simulink library "simetran"  (R2024b)
settings: Solver=VariableStepAuto  StartTime=0.0  StopTime=10.0  RelTol=1e-3
undefined symbols (not defined in the file): Csnu, gcbh, h, ResistanceM, Rsnu, Rt4, sps_rtmsupport, Ti, Ts, Z, Zm
libraries: fl_lib x81, nesl_utility x48, ee_lib x23
(part 2 of 3)

== system simetran/MATE_SSE_3Level/Subsystem2 ==
  g : Inport
  Capacitor : fl_lib/Electrical/Electrical Elements/Capacitor  c=SnubberCapacitance F  r=0 Ohm  g=0 1/Ohm  i_specify=off  i_priority=None  i=0 A  i_nominal_specify=off  i_nominal_value=1  i_nominal_unit=A  v_specify=off  v_priority=None  v=0 V  v_nominal_specify=off  v_nominal_value=1  v_nominal_unit=V  vc_specify=off  vc_priority=High  vc=0 V  vc_nominal_specify=off  vc_nominal_value=1  vc_nominal_unit=V
  Resistor : fl_lib/Electrical/Electrical Elements/Resistor  R=SnubberResistance Ohm  i_specify=off  i_priority=None  i=0 A  i_nominal_specify=off  i_nominal_value=1  i_nominal_unit=A  v_specify=off  v_priority=None  v=0 V  v_nominal_specify=off  v_nominal_value=1  v_nominal_unit=V
  SPST Switch : ee_lib/Switches & Breakers/SPST Switch  R_closed=Ron*2 Ohm  G_open=1e-6 S  Threshold=0.5 V  Width=0 V  model_dynamics=0  t_on=1e-3 s  t_off=1e-3 s  initial_vT=0 V
      settings: InternalSimscapePortConfiguration="{\"Bottom\":[],\"Left\":[{\"id\":\"vT\",\"label\":\"vT\",\"type\":\"input\"},{\"id\":\"p\",\"label\":\"\",\"type\":\"foundation.electrical.electrical\"}],\"Right\":[{\"id\":\"n\",\"label\":\"\",\"type\":\"foundation.electrical.electrical\"}],\"Top\":[]}"
  Simulink-PS Converter : nesl_utility/Simulink-PS Converter  PhysicalDomain=network_engine_domain  SubClassName=ps_input  LeftPortType=input  RightPortType=output  PseudoPeriodic=off  Frequencies=[]  NoiseDistribution=none  NoiseParameters=[]  Unit=1  AffineConversion=off  FilteringAndDerivatives=provide  SimscapeFilterOrder=1  InputFilterTimeConstant=0.001  UdotUserProvided=0
  P : PMIOPort  Side=Left
  N : PMIOPort  Port=2  Side=Right
  wires:
  g/1 -> Simulink-PS Converter/1
  connections:
  Capacitor/RConn1 -- Resistor/LConn1
  N/RConn1 -- Resistor/RConn1 -- SPST Switch/RConn1
  Simulink-PS Converter/RConn1 -- SPST Switch/LConn1
  P/RConn1 -- Capacitor/LConn1 -- SPST Switch/LConn2

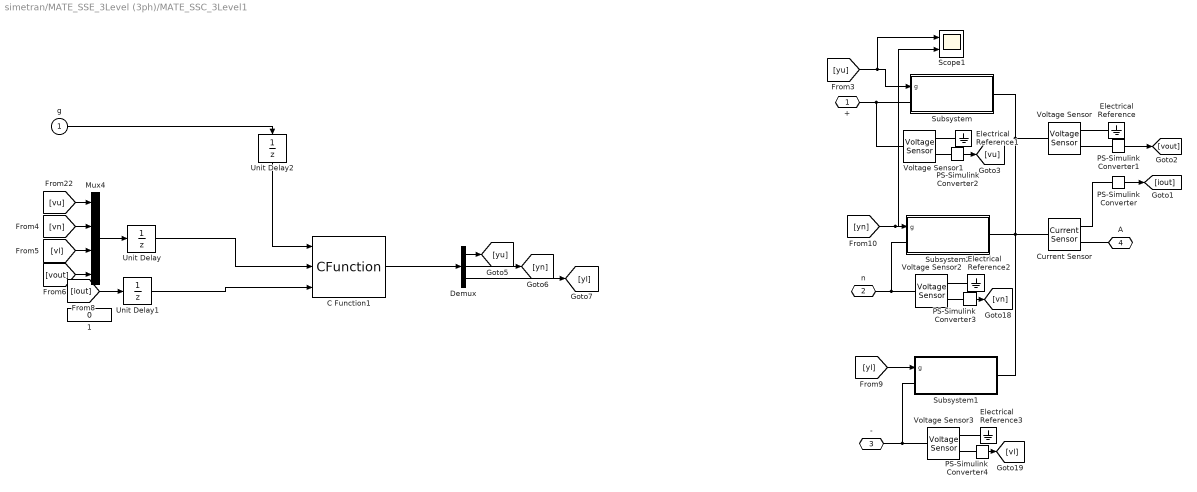
== system simetran/MATE_SSE_3Level (3ph)/MATE_SSC_3Level1 ==
  g : Inport
  1 : Constant  Value=0
  C Function1 : CFunction  OutputCode=|  InitializeConditionsCode=status_old=0;  CodegenOutputCode=|  CodegenInitializeConditionsCode=status_old=0;  CustomCodeSettingLocation=ModelConfigurationParameters
      OutputCode=|
      | {
      |     double status;
      | 
      |     //InputRealPtrsType gg      = ssGetInputPortRealSignalPtrs(S,0);
      |     //InputRealPtrsType Vtermm  = ssGetInputPortRealSignalPtrs(S,1);
      |     //InputRealPtrsType ioutt   = ssGetInputPortRealSignalPtrs(S,2);
      |     //InputRealPtrsType tol     = ssGetInputPortRealSignalPtrs(S,3);
      | 
      | 
      |     //real_T            *sw       =  ssGetOutputPortRealSignal(S,0);  // sw
      |     //real_T			  *stat     =  ssGetOutputPortRealSignal(S,1);  // status
      | 
      | 
      | 
      |     //mexPrintf("OUTPUTpause:\n");
      |     //mexEvalString("pause(2);");
      | 
      | 
      | 
      |     //real_T *status_old    = (real_T*) ssGetDWork(S,0);
      |     //real_T status[1];
      | 
      | 
      |     //real_T  g[4];
      |     //real_T  Vterm[4];
      |  
      | 
      |     //real_T iout[1];
      | 
      |    // *(g+0)= *gg[0];
      |    // *(g+1)= *gg[1];
      |    // *(g+2)= *gg[2];
      |    // *(g+3)= *gg[3];
      | 
      |    // *(Vterm+0)= *Vtermm[0];
      |    // *(Vterm+1)= *Vtermm[1];
      |    // *(Vterm+2)= *Vtermm[2];
      |    // *(Vterm+3)= *Vtermm[3];
      | 
      |    // iout= *ioutt[0];
      | 
      | 
      |  
      | 
      | 
      |     if (*(g+0)>0.5 && *(g+1)>0.5) {
      |         *(sw+0)=1;*(sw+1)=0;*(sw+2)=0;status=1;
      |     }
      |     else if (*(g+2)>0.5  && *(g+3)>0.5) {
      |         *(sw+0)=0;*(sw+1)=0;*(sw+2)=1;status=2;
      |     }
      |     else if (*(g+1)>0.5  && *(g+2)>0.5) {
      |         *(sw+0)=0;*(sw+1)=1;*(sw+2)=0;status=3;
      |     }
      |     else if (*(g+1)>0.5 && iout>0) {
      |         *(sw+0)=0;*(sw+1)=1;*(sw+2)=0;status=4;
      |     }
      |     else if (*(g+2)>0.5 && iout<0) {
      |         *(sw+0)=0;*(sw+1)=1;*(sw+2)=0;status=5;
      |     }
      |     else if ( (iout>0 && status_old<=6)) { //|| (*(iout>tol[0] && status_old>5) )  {
      |         *(sw+0)=0;*(sw+1)=0;*(sw+2)=1;status=6;
      |     }
      |     else if ( (iout<0 && status_old<=5) || (iout<0 && status_old==7) ) { // || (iout<(0-tol[0]) && status_old[0]>5)   ) {
      |         *(sw+0)=1;*(sw+1)=0;*(sw+2)=0;status=7;
      |     }
      |     else if ( (*(Vterm+3)>*(Vterm+1) && *(g+2)>0.5) || (*(Vterm+3)<*(Vterm+1)  && *(g+1)>0.5) ) {
      |         *(sw+0)=0;*(sw+1)=1;*(sw+2)=0;status=8;
      |     }
      |     else if (*(Vterm+3)>*(Vterm+0)) {
      |         *(sw+0)=1;*(sw+1)=0;*(sw+2)=0;status=9;
      |     }
      |     else if (*(Vterm+3)<*(Vterm+2)) {
      |         *(sw+0)=0;*(sw+1)=0;*(sw+2)=1;status=10;
      |     }
      |     else {
      |         *(sw+0)=0;*(sw+1)=0;*(sw+2)=0;status=11;
      |     }
      | 
      | 
      | 
      |     status_old=status;
      | 
      | 
      | }
      CodegenOutputCode=|
      | {
      |     double status;
      | 
      |     //InputRealPtrsType gg      = ssGetInputPortRealSignalPtrs(S,0);
      |     //InputRealPtrsType Vtermm  = ssGetInputPortRealSignalPtrs(S,1);
      |     //InputRealPtrsType ioutt   = ssGetInputPortRealSignalPtrs(S,2);
      |     //InputRealPtrsType tol     = ssGetInputPortRealSignalPtrs(S,3);
      | 
      | 
      |     //real_T            *sw       =  ssGetOutputPortRealSignal(S,0);  // sw
      |     //real_T			  *stat     =  ssGetOutputPortRealSignal(S,1);  // status
      | 
      | 
      | 
      |     //mexPrintf("OUTPUTpause:\n");
      |     //mexEvalString("pause(2);");
      | 
      | 
      | 
      |     //real_T *status_old    = (real_T*) ssGetDWork(S,0);
      |     //real_T status[1];
      | 
      | 
      |     //real_T  g[4];
      |     //real_T  Vterm[4];
      |  
      | 
      |     //real_T iout[1];
      | 
      |    // *(g+0)= *gg[0];
      |    // *(g+1)= *gg[1];
      |    // *(g+2)= *gg[2];
      |    // *(g+3)= *gg[3];
      | 
      |    // *(Vterm+0)= *Vtermm[0];
      |    // *(Vterm+1)= *Vtermm[1];
      |    // *(Vterm+2)= *Vtermm[2];
      |    // *(Vterm+3)= *Vtermm[3];
      | 
      |    // iout= *ioutt[0];
      | 
      | 
      |  
      | 
      | 
      |     if (*(g+0)>0.5 && *(g+1)>0.5) {
      |         *(sw+0)=1;*(sw+1)=0;*(sw+2)=0;status=1;
      |     }
      |     else if (*(g+2)>0.5  && *(g+3)>0.5) {
      |         *(sw+0)=0;*(sw+1)=0;*(sw+2)=1;status=2;
      |     }
      |     else if (*(g+1)>0.5  && *(g+2)>0.5) {
      |         *(sw+0)=0;*(sw+1)=1;*(sw+2)=0;status=3;
      |     }
      |     else if (*(g+1)>0.5 && iout>0) {
      |         *(sw+0)=0;*(sw+1)=1;*(sw+2)=0;status=4;
      |     }
      |     else if (*(g+2)>0.5 && iout<0) {
      |         *(sw+0)=0;*(sw+1)=1;*(sw+2)=0;status=5;
      |     }
      |     else if ( (iout>0 && status_old<=6)) { //|| (*(iout>tol[0] && status_old>5) )  {
      |         *(sw+0)=0;*(sw+1)=0;*(sw+2)=1;status=6;
      |     }
      |     else if ( (iout<0 && status_old<=5) || (iout<0 && status_old==7) ) { // || (iout<(0-tol[0]) && status_old[0]>5)   ) {
      |         *(sw+0)=1;*(sw+1)=0;*(sw+2)=0;status=7;
      |     }
      |     else if ( (*(Vterm+3)>*(Vterm+1) && *(g+2)>0.5) || (*(Vterm+3)<*(Vterm+1)  && *(g+1)>0.5) ) {
      |         *(sw+0)=0;*(sw+1)=1;*(sw+2)=0;status=8;
      |     }
      |     else if (*(Vterm+3)>*(Vterm+0)) {
      |         *(sw+0)=1;*(sw+1)=0;*(sw+2)=0;status=9;
      |     }
      |     else if (*(Vterm+3)<*(Vterm+2)) {
      |         *(sw+0)=0;*(sw+1)=0;*(sw+2)=1;status=10;
      |     }
      |     else {
      |         *(sw+0)=0;*(sw+1)=0;*(sw+2)=0;status=11;
      |     }
      | 
      | 
      | 
      |     status_old=status;
      | 
      | 
      | }
  Current Sensor : fl_lib/Electrical/Electrical Sensors/Current Sensor
  Demux : Demux  Outputs=3
  Electrical Reference{,1..3} (4 alike) : fl_lib/Electrical/Electrical Elements/Electrical Reference
  Mux4 : Mux
  PS-Simulink Converter{,1..4} (5 alike) : nesl_utility/PS-Simulink Converter  PhysicalDomain=network_engine_domain  SubClassName=ps_output  LeftPortType=input  RightPortType=output  PseudoPeriodic=off  Frequencies=[]  VectorFormat=inherit  Unit=inherit  AffineConversion=off
  Scope1 : Scope  NumInputPorts=2
  Subsystem : Subsystem
  Subsystem1 : Subsystem
  Subsystem2 : Subsystem
  Unit Delay : UnitDelay  SampleTime=Ts  HasFrameUpgradeWarning=on
  Unit Delay1 : UnitDelay  SampleTime=Ts  HasFrameUpgradeWarning=on
  Unit Delay2 : UnitDelay  SampleTime=Ts  HasFrameUpgradeWarning=on
  Voltage Sensor{,1..3} (4 alike) : fl_lib/Electrical/Electrical Sensors/Voltage Sensor
  + : PMIOPort  Side=Left
  n : PMIOPort  Port=2  Side=Left
  - : PMIOPort  Port=3  Side=Left
  A : PMIOPort  Port=4  Side=Right
  wires:
  Mux4/1 -> Unit Delay/1
  Demux/2 -> [yn]
  [vu] -> Mux4/1
  [vn] -> Mux4/2
  [vl] -> Mux4/3
  [vout] -> Mux4/4
  g/1 -> Unit Delay2/1
  Demux/3 -> [yl]
  Demux/1 -> [yu]
  [yu] -> Scope1/1, Subsystem/1(g)
  [yl] -> Subsystem1/1(g)
  [yn] -> Subsystem2/1(g), Scope1/2
  PS-Simulink Converter/1 -> [iout]
  PS-Simulink Converter1/1 -> [vout]
  PS-Simulink Converter2/1 -> [vu]
  PS-Simulink Converter3/1 -> [vn]
  PS-Simulink Converter4/1 -> [vl]
  [iout] -> Unit Delay1/1
  C Function1/1 -> Demux/1
  Unit Delay/1 -> C Function1/2
  Unit Delay1/1 -> C Function1/3
  Unit Delay2/1 -> C Function1/1
  connections:
  +/RConn1 -- Subsystem/LConn1 -- Voltage Sensor1/LConn1
  -/RConn1 -- Subsystem1/LConn1 -- Voltage Sensor3/LConn1
  Current Sensor/LConn1 -- Subsystem1/RConn1 -- Subsystem2/RConn1 -- Subsystem/RConn1 -- Voltage Sensor/LConn1
  n/RConn1 -- Subsystem2/LConn1 -- Voltage Sensor2/LConn1
  A/RConn1 -- Current Sensor/RConn2
  PS-Simulink Converter/LConn1 -- Current Sensor/RConn1
  Voltage Sensor/RConn2 -- Electrical Reference/LConn1
  Voltage Sensor/RConn1 -- PS-Simulink Converter1/LConn1
  Voltage Sensor1/RConn2 -- Electrical Reference1/LConn1
  Voltage Sensor1/RConn1 -- PS-Simulink Converter2/LConn1
  Voltage Sensor2/RConn1 -- PS-Simulink Converter3/LConn1
  Voltage Sensor2/RConn2 -- Electrical Reference2/LConn1
  Voltage Sensor3/RConn2 -- Electrical Reference3/LConn1
  Voltage Sensor3/RConn1 -- PS-Simulink Converter4/LConn1

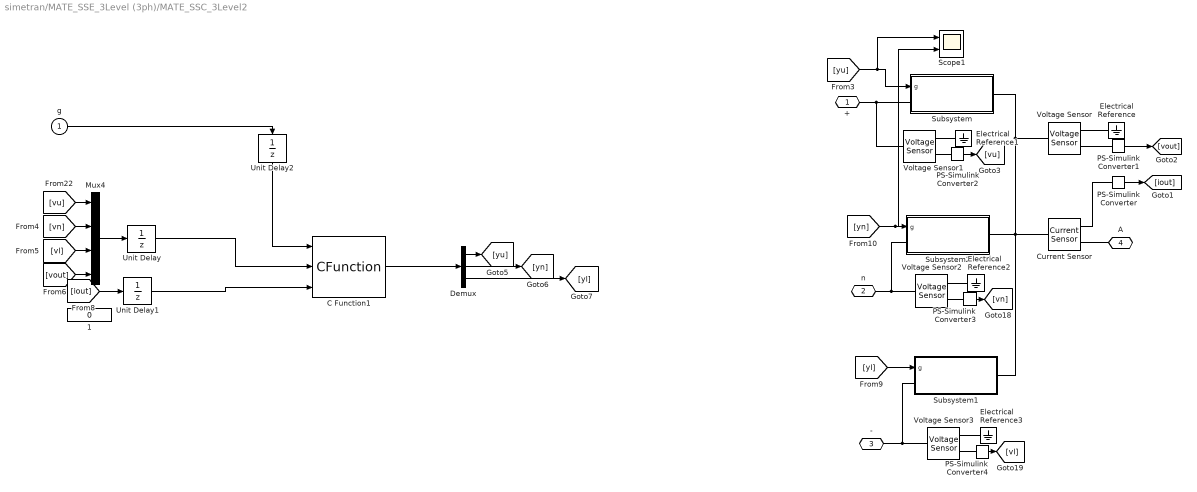
== system simetran/MATE_SSE_3Level (3ph)/MATE_SSC_3Level2 ==
  g : Inport
  1 : Constant  Value=0
  C Function1 : CFunction  OutputCode=|  InitializeConditionsCode=status_old=0;  CodegenOutputCode=|  CodegenInitializeConditionsCode=status_old=0;  CustomCodeSettingLocation=ModelConfigurationParameters
      OutputCode=|
      | {
      |     double status;
      | 
      |     //InputRealPtrsType gg      = ssGetInputPortRealSignalPtrs(S,0);
      |     //InputRealPtrsType Vtermm  = ssGetInputPortRealSignalPtrs(S,1);
      |     //InputRealPtrsType ioutt   = ssGetInputPortRealSignalPtrs(S,2);
      |     //InputRealPtrsType tol     = ssGetInputPortRealSignalPtrs(S,3);
      | 
      | 
      |     //real_T            *sw       =  ssGetOutputPortRealSignal(S,0);  // sw
      |     //real_T			  *stat     =  ssGetOutputPortRealSignal(S,1);  // status
      | 
      | 
      | 
      |     //mexPrintf("OUTPUTpause:\n");
      |     //mexEvalString("pause(2);");
      | 
      | 
      | 
      |     //real_T *status_old    = (real_T*) ssGetDWork(S,0);
      |     //real_T status[1];
      | 
      | 
      |     //real_T  g[4];
      |     //real_T  Vterm[4];
      |  
      | 
      |     //real_T iout[1];
      | 
      |    // *(g+0)= *gg[0];
      |    // *(g+1)= *gg[1];
      |    // *(g+2)= *gg[2];
      |    // *(g+3)= *gg[3];
      | 
      |    // *(Vterm+0)= *Vtermm[0];
      |    // *(Vterm+1)= *Vtermm[1];
      |    // *(Vterm+2)= *Vtermm[2];
      |    // *(Vterm+3)= *Vtermm[3];
      | 
      |    // iout= *ioutt[0];
      | 
      | 
      |  
      | 
      | 
      |     if (*(g+0)>0.5 && *(g+1)>0.5) {
      |         *(sw+0)=1;*(sw+1)=0;*(sw+2)=0;status=1;
      |     }
      |     else if (*(g+2)>0.5  && *(g+3)>0.5) {
      |         *(sw+0)=0;*(sw+1)=0;*(sw+2)=1;status=2;
      |     }
      |     else if (*(g+1)>0.5  && *(g+2)>0.5) {
      |         *(sw+0)=0;*(sw+1)=1;*(sw+2)=0;status=3;
      |     }
      |     else if (*(g+1)>0.5 && iout>0) {
      |         *(sw+0)=0;*(sw+1)=1;*(sw+2)=0;status=4;
      |     }
      |     else if (*(g+2)>0.5 && iout<0) {
      |         *(sw+0)=0;*(sw+1)=1;*(sw+2)=0;status=5;
      |     }
      |     else if ( (iout>0 && status_old<=6)) { //|| (*(iout>tol[0] && status_old>5) )  {
      |         *(sw+0)=0;*(sw+1)=0;*(sw+2)=1;status=6;
      |     }
      |     else if ( (iout<0 && status_old<=5) || (iout<0 && status_old==7) ) { // || (iout<(0-tol[0]) && status_old[0]>5)   ) {
      |         *(sw+0)=1;*(sw+1)=0;*(sw+2)=0;status=7;
      |     }
      |     else if ( (*(Vterm+3)>*(Vterm+1) && *(g+2)>0.5) || (*(Vterm+3)<*(Vterm+1)  && *(g+1)>0.5) ) {
      |         *(sw+0)=0;*(sw+1)=1;*(sw+2)=0;status=8;
      |     }
      |     else if (*(Vterm+3)>*(Vterm+0)) {
      |         *(sw+0)=1;*(sw+1)=0;*(sw+2)=0;status=9;
      |     }
      |     else if (*(Vterm+3)<*(Vterm+2)) {
      |         *(sw+0)=0;*(sw+1)=0;*(sw+2)=1;status=10;
      |     }
      |     else {
      |         *(sw+0)=0;*(sw+1)=0;*(sw+2)=0;status=11;
      |     }
      | 
      | 
      | 
      |     status_old=status;
      | 
      | 
      | }
      CodegenOutputCode=|
      | {
      |     double status;
      | 
      |     //InputRealPtrsType gg      = ssGetInputPortRealSignalPtrs(S,0);
      |     //InputRealPtrsType Vtermm  = ssGetInputPortRealSignalPtrs(S,1);
      |     //InputRealPtrsType ioutt   = ssGetInputPortRealSignalPtrs(S,2);
      |     //InputRealPtrsType tol     = ssGetInputPortRealSignalPtrs(S,3);
      | 
      | 
      |     //real_T            *sw       =  ssGetOutputPortRealSignal(S,0);  // sw
      |     //real_T			  *stat     =  ssGetOutputPortRealSignal(S,1);  // status
      | 
      | 
      | 
      |     //mexPrintf("OUTPUTpause:\n");
      |     //mexEvalString("pause(2);");
      | 
      | 
      | 
      |     //real_T *status_old    = (real_T*) ssGetDWork(S,0);
      |     //real_T status[1];
      | 
      | 
      |     //real_T  g[4];
      |     //real_T  Vterm[4];
      |  
      | 
      |     //real_T iout[1];
      | 
      |    // *(g+0)= *gg[0];
      |    // *(g+1)= *gg[1];
      |    // *(g+2)= *gg[2];
      |    // *(g+3)= *gg[3];
      | 
      |    // *(Vterm+0)= *Vtermm[0];
      |    // *(Vterm+1)= *Vtermm[1];
      |    // *(Vterm+2)= *Vtermm[2];
      |    // *(Vterm+3)= *Vtermm[3];
      | 
      |    // iout= *ioutt[0];
      | 
      | 
      |  
      | 
      | 
      |     if (*(g+0)>0.5 && *(g+1)>0.5) {
      |         *(sw+0)=1;*(sw+1)=0;*(sw+2)=0;status=1;
      |     }
      |     else if (*(g+2)>0.5  && *(g+3)>0.5) {
      |         *(sw+0)=0;*(sw+1)=0;*(sw+2)=1;status=2;
      |     }
      |     else if (*(g+1)>0.5  && *(g+2)>0.5) {
      |         *(sw+0)=0;*(sw+1)=1;*(sw+2)=0;status=3;
      |     }
      |     else if (*(g+1)>0.5 && iout>0) {
      |         *(sw+0)=0;*(sw+1)=1;*(sw+2)=0;status=4;
      |     }
      |     else if (*(g+2)>0.5 && iout<0) {
      |         *(sw+0)=0;*(sw+1)=1;*(sw+2)=0;status=5;
      |     }
      |     else if ( (iout>0 && status_old<=6)) { //|| (*(iout>tol[0] && status_old>5) )  {
      |         *(sw+0)=0;*(sw+1)=0;*(sw+2)=1;status=6;
      |     }
      |     else if ( (iout<0 && status_old<=5) || (iout<0 && status_old==7) ) { // || (iout<(0-tol[0]) && status_old[0]>5)   ) {
      |         *(sw+0)=1;*(sw+1)=0;*(sw+2)=0;status=7;
      |     }
      |     else if ( (*(Vterm+3)>*(Vterm+1) && *(g+2)>0.5) || (*(Vterm+3)<*(Vterm+1)  && *(g+1)>0.5) ) {
      |         *(sw+0)=0;*(sw+1)=1;*(sw+2)=0;status=8;
      |     }
      |     else if (*(Vterm+3)>*(Vterm+0)) {
      |         *(sw+0)=1;*(sw+1)=0;*(sw+2)=0;status=9;
      |     }
      |     else if (*(Vterm+3)<*(Vterm+2)) {
      |         *(sw+0)=0;*(sw+1)=0;*(sw+2)=1;status=10;
      |     }
      |     else {
      |         *(sw+0)=0;*(sw+1)=0;*(sw+2)=0;status=11;
      |     }
      | 
      | 
      | 
      |     status_old=status;
      | 
      | 
      | }
  Current Sensor : fl_lib/Electrical/Electrical Sensors/Current Sensor
  Demux : Demux  Outputs=3
  Electrical Reference{,1..3} (4 alike) : fl_lib/Electrical/Electrical Elements/Electrical Reference
  Mux4 : Mux
  PS-Simulink Converter{,1..4} (5 alike) : nesl_utility/PS-Simulink Converter  PhysicalDomain=network_engine_domain  SubClassName=ps_output  LeftPortType=input  RightPortType=output  PseudoPeriodic=off  Frequencies=[]  VectorFormat=inherit  Unit=inherit  AffineConversion=off
  Scope1 : Scope  NumInputPorts=2
  Subsystem : Subsystem
  Subsystem1 : Subsystem
  Subsystem2 : Subsystem
  Unit Delay : UnitDelay  SampleTime=Ts  HasFrameUpgradeWarning=on
  Unit Delay1 : UnitDelay  SampleTime=Ts  HasFrameUpgradeWarning=on
  Unit Delay2 : UnitDelay  SampleTime=Ts  HasFrameUpgradeWarning=on
  Voltage Sensor{,1..3} (4 alike) : fl_lib/Electrical/Electrical Sensors/Voltage Sensor
  + : PMIOPort  Side=Left
  n : PMIOPort  Port=2  Side=Left
  - : PMIOPort  Port=3  Side=Left
  A : PMIOPort  Port=4  Side=Right
  wires:
  Mux4/1 -> Unit Delay/1
  Demux/2 -> [yn]
  [vu] -> Mux4/1
  [vn] -> Mux4/2
  [vl] -> Mux4/3
  [vout] -> Mux4/4
  g/1 -> Unit Delay2/1
  Demux/3 -> [yl]
  Demux/1 -> [yu]
  [yu] -> Scope1/1, Subsystem/1(g)
  [yl] -> Subsystem1/1(g)
  [yn] -> Subsystem2/1(g), Scope1/2
  PS-Simulink Converter/1 -> [iout]
  PS-Simulink Converter1/1 -> [vout]
  PS-Simulink Converter2/1 -> [vu]
  PS-Simulink Converter3/1 -> [vn]
  PS-Simulink Converter4/1 -> [vl]
  [iout] -> Unit Delay1/1
  C Function1/1 -> Demux/1
  Unit Delay/1 -> C Function1/2
  Unit Delay1/1 -> C Function1/3
  Unit Delay2/1 -> C Function1/1
  connections:
  +/RConn1 -- Subsystem/LConn1 -- Voltage Sensor1/LConn1
  -/RConn1 -- Subsystem1/LConn1 -- Voltage Sensor3/LConn1
  Current Sensor/LConn1 -- Subsystem1/RConn1 -- Subsystem2/RConn1 -- Subsystem/RConn1 -- Voltage Sensor/LConn1
  n/RConn1 -- Subsystem2/LConn1 -- Voltage Sensor2/LConn1
  A/RConn1 -- Current Sensor/RConn2
  PS-Simulink Converter/LConn1 -- Current Sensor/RConn1
  Voltage Sensor/RConn2 -- Electrical Reference/LConn1
  Voltage Sensor/RConn1 -- PS-Simulink Converter1/LConn1
  Voltage Sensor1/RConn2 -- Electrical Reference1/LConn1
  Voltage Sensor1/RConn1 -- PS-Simulink Converter2/LConn1
  Voltage Sensor2/RConn1 -- PS-Simulink Converter3/LConn1
  Voltage Sensor2/RConn2 -- Electrical Reference2/LConn1
  Voltage Sensor3/RConn2 -- Electrical Reference3/LConn1
  Voltage Sensor3/RConn1 -- PS-Simulink Converter4/LConn1

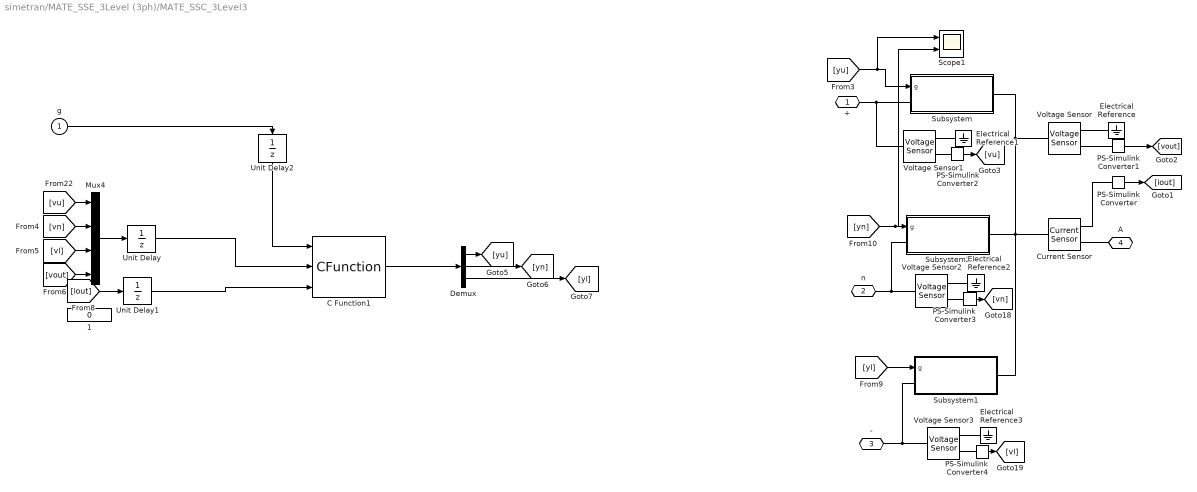
== system simetran/MATE_SSE_3Level (3ph)/MATE_SSC_3Level3 ==
  g : Inport
  1 : Constant  Value=0
  C Function1 : CFunction  OutputCode=|  InitializeConditionsCode=status_old=0;  CodegenOutputCode=|  CodegenInitializeConditionsCode=status_old=0;  CustomCodeSettingLocation=ModelConfigurationParameters
      OutputCode=|
      | {
      |     double status;
      | 
      |     //InputRealPtrsType gg      = ssGetInputPortRealSignalPtrs(S,0);
      |     //InputRealPtrsType Vtermm  = ssGetInputPortRealSignalPtrs(S,1);
      |     //InputRealPtrsType ioutt   = ssGetInputPortRealSignalPtrs(S,2);
      |     //InputRealPtrsType tol     = ssGetInputPortRealSignalPtrs(S,3);
      | 
      | 
      |     //real_T            *sw       =  ssGetOutputPortRealSignal(S,0);  // sw
      |     //real_T			  *stat     =  ssGetOutputPortRealSignal(S,1);  // status
      | 
      | 
      | 
      |     //mexPrintf("OUTPUTpause:\n");
      |     //mexEvalString("pause(2);");
      | 
      | 
      | 
      |     //real_T *status_old    = (real_T*) ssGetDWork(S,0);
      |     //real_T status[1];
      | 
      | 
      |     //real_T  g[4];
      |     //real_T  Vterm[4];
      |  
      | 
      |     //real_T iout[1];
      | 
      |    // *(g+0)= *gg[0];
      |    // *(g+1)= *gg[1];
      |    // *(g+2)= *gg[2];
      |    // *(g+3)= *gg[3];
      | 
      |    // *(Vterm+0)= *Vtermm[0];
      |    // *(Vterm+1)= *Vtermm[1];
      |    // *(Vterm+2)= *Vtermm[2];
      |    // *(Vterm+3)= *Vtermm[3];
      | 
      |    // iout= *ioutt[0];
      | 
      | 
      |  
      | 
      | 
      |     if (*(g+0)>0.5 && *(g+1)>0.5) {
      |         *(sw+0)=1;*(sw+1)=0;*(sw+2)=0;status=1;
      |     }
      |     else if (*(g+2)>0.5  && *(g+3)>0.5) {
      |         *(sw+0)=0;*(sw+1)=0;*(sw+2)=1;status=2;
      |     }
      |     else if (*(g+1)>0.5  && *(g+2)>0.5) {
      |         *(sw+0)=0;*(sw+1)=1;*(sw+2)=0;status=3;
      |     }
      |     else if (*(g+1)>0.5 && iout>0) {
      |         *(sw+0)=0;*(sw+1)=1;*(sw+2)=0;status=4;
      |     }
      |     else if (*(g+2)>0.5 && iout<0) {
      |         *(sw+0)=0;*(sw+1)=1;*(sw+2)=0;status=5;
      |     }
      |     else if ( (iout>0 && status_old<=6)) { //|| (*(iout>tol[0] && status_old>5) )  {
      |         *(sw+0)=0;*(sw+1)=0;*(sw+2)=1;status=6;
      |     }
      |     else if ( (iout<0 && status_old<=5) || (iout<0 && status_old==7) ) { // || (iout<(0-tol[0]) && status_old[0]>5)   ) {
      |         *(sw+0)=1;*(sw+1)=0;*(sw+2)=0;status=7;
      |     }
      |     else if ( (*(Vterm+3)>*(Vterm+1) && *(g+2)>0.5) || (*(Vterm+3)<*(Vterm+1)  && *(g+1)>0.5) ) {
      |         *(sw+0)=0;*(sw+1)=1;*(sw+2)=0;status=8;
      |     }
      |     else if (*(Vterm+3)>*(Vterm+0)) {
      |         *(sw+0)=1;*(sw+1)=0;*(sw+2)=0;status=9;
      |     }
      |     else if (*(Vterm+3)<*(Vterm+2)) {
      |         *(sw+0)=0;*(sw+1)=0;*(sw+2)=1;status=10;
      |     }
      |     else {
      |         *(sw+0)=0;*(sw+1)=0;*(sw+2)=0;status=11;
      |     }
      | 
      | 
      | 
      |     status_old=status;
      | 
      | 
      | }
      CodegenOutputCode=|
      | {
      |     double status;
      | 
      |     //InputRealPtrsType gg      = ssGetInputPortRealSignalPtrs(S,0);
      |     //InputRealPtrsType Vtermm  = ssGetInputPortRealSignalPtrs(S,1);
      |     //InputRealPtrsType ioutt   = ssGetInputPortRealSignalPtrs(S,2);
      |     //InputRealPtrsType tol     = ssGetInputPortRealSignalPtrs(S,3);
      | 
      | 
      |     //real_T            *sw       =  ssGetOutputPortRealSignal(S,0);  // sw
      |     //real_T			  *stat     =  ssGetOutputPortRealSignal(S,1);  // status
      | 
      | 
      | 
      |     //mexPrintf("OUTPUTpause:\n");
      |     //mexEvalString("pause(2);");
      | 
      | 
      | 
      |     //real_T *status_old    = (real_T*) ssGetDWork(S,0);
      |     //real_T status[1];
      | 
      | 
      |     //real_T  g[4];
      |     //real_T  Vterm[4];
      |  
      | 
      |     //real_T iout[1];
      | 
      |    // *(g+0)= *gg[0];
      |    // *(g+1)= *gg[1];
      |    // *(g+2)= *gg[2];
      |    // *(g+3)= *gg[3];
      | 
      |    // *(Vterm+0)= *Vtermm[0];
      |    // *(Vterm+1)= *Vtermm[1];
      |    // *(Vterm+2)= *Vtermm[2];
      |    // *(Vterm+3)= *Vtermm[3];
      | 
      |    // iout= *ioutt[0];
      | 
      | 
      |  
      | 
      | 
      |     if (*(g+0)>0.5 && *(g+1)>0.5) {
      |         *(sw+0)=1;*(sw+1)=0;*(sw+2)=0;status=1;
      |     }
      |     else if (*(g+2)>0.5  && *(g+3)>0.5) {
      |         *(sw+0)=0;*(sw+1)=0;*(sw+2)=1;status=2;
      |     }
      |     else if (*(g+1)>0.5  && *(g+2)>0.5) {
      |         *(sw+0)=0;*(sw+1)=1;*(sw+2)=0;status=3;
      |     }
      |     else if (*(g+1)>0.5 && iout>0) {
      |         *(sw+0)=0;*(sw+1)=1;*(sw+2)=0;status=4;
      |     }
      |     else if (*(g+2)>0.5 && iout<0) {
      |         *(sw+0)=0;*(sw+1)=1;*(sw+2)=0;status=5;
      |     }
      |     else if ( (iout>0 && status_old<=6)) { //|| (*(iout>tol[0] && status_old>5) )  {
      |         *(sw+0)=0;*(sw+1)=0;*(sw+2)=1;status=6;
      |     }
      |     else if ( (iout<0 && status_old<=5) || (iout<0 && status_old==7) ) { // || (iout<(0-tol[0]) && status_old[0]>5)   ) {
      |         *(sw+0)=1;*(sw+1)=0;*(sw+2)=0;status=7;
      |     }
      |     else if ( (*(Vterm+3)>*(Vterm+1) && *(g+2)>0.5) || (*(Vterm+3)<*(Vterm+1)  && *(g+1)>0.5) ) {
      |         *(sw+0)=0;*(sw+1)=1;*(sw+2)=0;status=8;
      |     }
      |     else if (*(Vterm+3)>*(Vterm+0)) {
      |         *(sw+0)=1;*(sw+1)=0;*(sw+2)=0;status=9;
      |     }
      |     else if (*(Vterm+3)<*(Vterm+2)) {
      |         *(sw+0)=0;*(sw+1)=0;*(sw+2)=1;status=10;
      |     }
      |     else {
      |         *(sw+0)=0;*(sw+1)=0;*(sw+2)=0;status=11;
      |     }
      | 
      | 
      | 
      |     status_old=status;
      | 
      | 
      | }
  Current Sensor : fl_lib/Electrical/Electrical Sensors/Current Sensor
  Demux : Demux  Outputs=3
  Electrical Reference{,1..3} (4 alike) : fl_lib/Electrical/Electrical Elements/Electrical Reference
  Mux4 : Mux
  PS-Simulink Converter{,1..4} (5 alike) : nesl_utility/PS-Simulink Converter  PhysicalDomain=network_engine_domain  SubClassName=ps_output  LeftPortType=input  RightPortType=output  PseudoPeriodic=off  Frequencies=[]  VectorFormat=inherit  Unit=inherit  AffineConversion=off
  Scope1 : Scope  NumInputPorts=2
  Subsystem : Subsystem
  Subsystem1 : Subsystem
  Subsystem2 : Subsystem
  Unit Delay : UnitDelay  SampleTime=Ts  HasFrameUpgradeWarning=on
  Unit Delay1 : UnitDelay  SampleTime=Ts  HasFrameUpgradeWarning=on
  Unit Delay2 : UnitDelay  SampleTime=Ts  HasFrameUpgradeWarning=on
  Voltage Sensor{,1..3} (4 alike) : fl_lib/Electrical/Electrical Sensors/Voltage Sensor
  + : PMIOPort  Side=Left
  n : PMIOPort  Port=2  Side=Left
  - : PMIOPort  Port=3  Side=Left
  A : PMIOPort  Port=4  Side=Right
  wires:
  Mux4/1 -> Unit Delay/1
  Demux/2 -> [yn]
  [vu] -> Mux4/1
  [vn] -> Mux4/2
  [vl] -> Mux4/3
  [vout] -> Mux4/4
  g/1 -> Unit Delay2/1
  Demux/3 -> [yl]
  Demux/1 -> [yu]
  [yu] -> Scope1/1, Subsystem/1(g)
  [yl] -> Subsystem1/1(g)
  [yn] -> Subsystem2/1(g), Scope1/2
  PS-Simulink Converter/1 -> [iout]
  PS-Simulink Converter1/1 -> [vout]
  PS-Simulink Converter2/1 -> [vu]
  PS-Simulink Converter3/1 -> [vn]
  PS-Simulink Converter4/1 -> [vl]
  [iout] -> Unit Delay1/1
  C Function1/1 -> Demux/1
  Unit Delay/1 -> C Function1/2
  Unit Delay1/1 -> C Function1/3
  Unit Delay2/1 -> C Function1/1
  connections:
  +/RConn1 -- Subsystem/LConn1 -- Voltage Sensor1/LConn1
  -/RConn1 -- Subsystem1/LConn1 -- Voltage Sensor3/LConn1
  Current Sensor/LConn1 -- Subsystem1/RConn1 -- Subsystem2/RConn1 -- Subsystem/RConn1 -- Voltage Sensor/LConn1
  n/RConn1 -- Subsystem2/LConn1 -- Voltage Sensor2/LConn1
  A/RConn1 -- Current Sensor/RConn2
  PS-Simulink Converter/LConn1 -- Current Sensor/RConn1
  Voltage Sensor/RConn2 -- Electrical Reference/LConn1
  Voltage Sensor/RConn1 -- PS-Simulink Converter1/LConn1
  Voltage Sensor1/RConn2 -- Electrical Reference1/LConn1
  Voltage Sensor1/RConn1 -- PS-Simulink Converter2/LConn1
  Voltage Sensor2/RConn1 -- PS-Simulink Converter3/LConn1
  Voltage Sensor2/RConn2 -- Electrical Reference2/LConn1
  Voltage Sensor3/RConn2 -- Electrical Reference3/LConn1
  Voltage Sensor3/RConn1 -- PS-Simulink Converter4/LConn1

== system simetran/RTScapeHalfStub/SL1 ==
  i : Inport
  demistub : Subsystem
  + : PMIOPort  Side=Left
  - : PMIOPort  Port=2  Side=Right
  o : Outport  VectorParamsAs1DForOutWhenUnconnected=off
  wires:
  i/1 -> demistub/1(hist_in)
  demistub/1(hist_out) -> o/1
  connections:
  +/RConn1 -- demistub/LConn1
  -/RConn1 -- demistub/LConn2

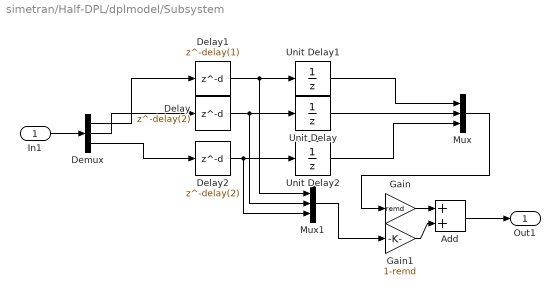
== system simetran/Half-DPL/dplmodel/Subsystem ==
  In1 : Inport
  Add : Sum
  Delay : Delay  DelayLength=delay(2)
  Delay1 : Delay  DelayLength=delay(1)
  Delay2 : Delay  DelayLength=delay(2)
  Demux : Demux  Outputs=3
  Gain : Gain  Gain=remd
  Gain1 : Gain  Gain=1-remd
  Mux : Mux  Inputs=3
  Mux1 : Mux  Inputs=3
  Unit Delay : UnitDelay  SampleTime=Ts  HasFrameUpgradeWarning=on
  Unit Delay1 : UnitDelay  SampleTime=Ts  HasFrameUpgradeWarning=on
  Unit Delay2 : UnitDelay  SampleTime=Ts  HasFrameUpgradeWarning=on
  Out1 : Outport
  wires:
  In1/1 -> Demux/1
  Demux/2 -> Delay/1
  Demux/3 -> Delay2/1
  Demux/1 -> Delay1/1
  Delay1/1 -> Mux1/1, Unit Delay1/1
  Delay/1 -> Mux1/2, Unit Delay/1
  Delay2/1 -> Mux1/3, Unit Delay2/1
  Gain/1 -> Add/1
  Gain1/1 -> Add/2
  Unit Delay/1 -> Mux/2
  Unit Delay1/1 -> Mux/1
  Unit Delay2/1 -> Mux/3
  Add/1 -> Out1/1
  Mux/1 -> Gain/1
  Mux1/1 -> Gain1/1

== system simetran/MATE_SSE_3Level (3ph)/MATE_SSC_3Level1/Subsystem ==
  g : Inport
  Capacitor : fl_lib/Electrical/Electrical Elements/Capacitor  c=SnubberCapacitance F  r=0 Ohm  g=0 1/Ohm  i_specify=off  i_priority=None  i=0 A  i_nominal_specify=off  i_nominal_value=1  i_nominal_unit=A  v_specify=off  v_priority=None  v=0 V  v_nominal_specify=off  v_nominal_value=1  v_nominal_unit=V  vc_specify=off  vc_priority=High  vc=0 V  vc_nominal_specify=off  vc_nominal_value=1  vc_nominal_unit=V
  Resistor : fl_lib/Electrical/Electrical Elements/Resistor  R=SnubberResistance Ohm  i_specify=off  i_priority=None  i=0 A  i_nominal_specify=off  i_nominal_value=1  i_nominal_unit=A  v_specify=off  v_priority=None  v=0 V  v_nominal_specify=off  v_nominal_value=1  v_nominal_unit=V
  SPST Switch : ee_lib/Switches & Breakers/SPST Switch  R_closed=Ron*2 Ohm  G_open=1e-6 S  Threshold=0.5 V  Width=0 V  model_dynamics=0  t_on=1e-3 s  t_off=1e-3 s  initial_vT=0 V
      settings: InternalSimscapePortConfiguration="{\"Bottom\":[],\"Left\":[{\"id\":\"vT\",\"label\":\"vT\",\"type\":\"input\"},{\"id\":\"p\",\"label\":\"\",\"type\":\"foundation.electrical.electrical\"}],\"Right\":[{\"id\":\"n\",\"label\":\"\",\"type\":\"foundation.electrical.electrical\"}],\"Top\":[]}"
  Simulink-PS Converter : nesl_utility/Simulink-PS Converter  PhysicalDomain=network_engine_domain  SubClassName=ps_input  LeftPortType=input  RightPortType=output  PseudoPeriodic=off  Frequencies=[]  NoiseDistribution=none  NoiseParameters=[]  Unit=1  AffineConversion=off  FilteringAndDerivatives=provide  SimscapeFilterOrder=1  InputFilterTimeConstant=0.001  UdotUserProvided=0
  P : PMIOPort  Side=Left
  N : PMIOPort  Port=2  Side=Right
  wires:
  g/1 -> Simulink-PS Converter/1
  connections:
  SPST Switch/LConn2 -- Capacitor/LConn1 -- P/RConn1
  Simulink-PS Converter/RConn1 -- SPST Switch/LConn1
  SPST Switch/RConn1 -- Resistor/RConn1 -- N/RConn1
  Capacitor/RConn1 -- Resistor/LConn1

== system simetran/MATE_SSE_3Level (3ph)/MATE_SSC_3Level1/Subsystem1 ==
  g : Inport
  Capacitor : fl_lib/Electrical/Electrical Elements/Capacitor  c=SnubberCapacitance F  r=0 Ohm  g=0 1/Ohm  i_specify=off  i_priority=None  i=0 A  i_nominal_specify=off  i_nominal_value=1  i_nominal_unit=A  v_specify=off  v_priority=None  v=0 V  v_nominal_specify=off  v_nominal_value=1  v_nominal_unit=V  vc_specify=off  vc_priority=High  vc=0 V  vc_nominal_specify=off  vc_nominal_value=1  vc_nominal_unit=V
  Resistor : fl_lib/Electrical/Electrical Elements/Resistor  R=SnubberResistance Ohm  i_specify=off  i_priority=None  i=0 A  i_nominal_specify=off  i_nominal_value=1  i_nominal_unit=A  v_specify=off  v_priority=None  v=0 V  v_nominal_specify=off  v_nominal_value=1  v_nominal_unit=V
  SPST Switch : ee_lib/Switches & Breakers/SPST Switch  R_closed=Ron*2 Ohm  G_open=1e-6 S  Threshold=0.5 V  Width=0 V  model_dynamics=0  t_on=1e-3 s  t_off=1e-3 s  initial_vT=0 V
      settings: InternalSimscapePortConfiguration="{\"Bottom\":[],\"Left\":[{\"id\":\"vT\",\"label\":\"vT\",\"type\":\"input\"},{\"id\":\"p\",\"label\":\"\",\"type\":\"foundation.electrical.electrical\"}],\"Right\":[{\"id\":\"n\",\"label\":\"\",\"type\":\"foundation.electrical.electrical\"}],\"Top\":[]}"
  Simulink-PS Converter : nesl_utility/Simulink-PS Converter  PhysicalDomain=network_engine_domain  SubClassName=ps_input  LeftPortType=input  RightPortType=output  PseudoPeriodic=off  Frequencies=[]  NoiseDistribution=none  NoiseParameters=[]  Unit=1  AffineConversion=off  FilteringAndDerivatives=provide  SimscapeFilterOrder=1  InputFilterTimeConstant=0.001  UdotUserProvided=0
  P : PMIOPort  Side=Left
  N : PMIOPort  Port=2  Side=Right
  wires:
  g/1 -> Simulink-PS Converter/1
  connections:
  SPST Switch/LConn2 -- Capacitor/LConn1 -- P/RConn1
  Simulink-PS Converter/RConn1 -- SPST Switch/LConn1
  SPST Switch/RConn1 -- Resistor/RConn1 -- N/RConn1
  Capacitor/RConn1 -- Resistor/LConn1

== system simetran/MATE_SSE_3Level (3ph)/MATE_SSC_3Level1/Subsystem2 ==
  g : Inport
  Capacitor : fl_lib/Electrical/Electrical Elements/Capacitor  c=SnubberCapacitance F  r=0 Ohm  g=0 1/Ohm  i_specify=off  i_priority=None  i=0 A  i_nominal_specify=off  i_nominal_value=1  i_nominal_unit=A  v_specify=off  v_priority=None  v=0 V  v_nominal_specify=off  v_nominal_value=1  v_nominal_unit=V  vc_specify=off  vc_priority=High  vc=0 V  vc_nominal_specify=off  vc_nominal_value=1  vc_nominal_unit=V
  Resistor : fl_lib/Electrical/Electrical Elements/Resistor  R=SnubberResistance Ohm  i_specify=off  i_priority=None  i=0 A  i_nominal_specify=off  i_nominal_value=1  i_nominal_unit=A  v_specify=off  v_priority=None  v=0 V  v_nominal_specify=off  v_nominal_value=1  v_nominal_unit=V
  SPST Switch : ee_lib/Switches & Breakers/SPST Switch  R_closed=Ron*2 Ohm  G_open=1e-6 S  Threshold=0.5 V  Width=0 V  model_dynamics=0  t_on=1e-3 s  t_off=1e-3 s  initial_vT=0 V
      settings: InternalSimscapePortConfiguration="{\"Bottom\":[],\"Left\":[{\"id\":\"vT\",\"label\":\"vT\",\"type\":\"input\"},{\"id\":\"p\",\"label\":\"\",\"type\":\"foundation.electrical.electrical\"}],\"Right\":[{\"id\":\"n\",\"label\":\"\",\"type\":\"foundation.electrical.electrical\"}],\"Top\":[]}"
  Simulink-PS Converter : nesl_utility/Simulink-PS Converter  PhysicalDomain=network_engine_domain  SubClassName=ps_input  LeftPortType=input  RightPortType=output  PseudoPeriodic=off  Frequencies=[]  NoiseDistribution=none  NoiseParameters=[]  Unit=1  AffineConversion=off  FilteringAndDerivatives=provide  SimscapeFilterOrder=1  InputFilterTimeConstant=0.001  UdotUserProvided=0
  P : PMIOPort  Side=Left
  N : PMIOPort  Port=2  Side=Right
  wires:
  g/1 -> Simulink-PS Converter/1
  connections:
  Capacitor/RConn1 -- Resistor/LConn1
  N/RConn1 -- Resistor/RConn1 -- SPST Switch/RConn1
  Simulink-PS Converter/RConn1 -- SPST Switch/LConn1
  P/RConn1 -- Capacitor/LConn1 -- SPST Switch/LConn2

== system simetran/MATE_SSE_3Level (3ph)/MATE_SSC_3Level2/Subsystem ==
  g : Inport
  Capacitor : fl_lib/Electrical/Electrical Elements/Capacitor  c=SnubberCapacitance F  r=0 Ohm  g=0 1/Ohm  i_specify=off  i_priority=None  i=0 A  i_nominal_specify=off  i_nominal_value=1  i_nominal_unit=A  v_specify=off  v_priority=None  v=0 V  v_nominal_specify=off  v_nominal_value=1  v_nominal_unit=V  vc_specify=off  vc_priority=High  vc=0 V  vc_nominal_specify=off  vc_nominal_value=1  vc_nominal_unit=V
  Resistor : fl_lib/Electrical/Electrical Elements/Resistor  R=SnubberResistance Ohm  i_specify=off  i_priority=None  i=0 A  i_nominal_specify=off  i_nominal_value=1  i_nominal_unit=A  v_specify=off  v_priority=None  v=0 V  v_nominal_specify=off  v_nominal_value=1  v_nominal_unit=V
  SPST Switch : ee_lib/Switches & Breakers/SPST Switch  R_closed=Ron*2 Ohm  G_open=1e-6 S  Threshold=0.5 V  Width=0 V  model_dynamics=0  t_on=1e-3 s  t_off=1e-3 s  initial_vT=0 V
      settings: InternalSimscapePortConfiguration="{\"Bottom\":[],\"Left\":[{\"id\":\"vT\",\"label\":\"vT\",\"type\":\"input\"},{\"id\":\"p\",\"label\":\"\",\"type\":\"foundation.electrical.electrical\"}],\"Right\":[{\"id\":\"n\",\"label\":\"\",\"type\":\"foundation.electrical.electrical\"}],\"Top\":[]}"
  Simulink-PS Converter : nesl_utility/Simulink-PS Converter  PhysicalDomain=network_engine_domain  SubClassName=ps_input  LeftPortType=input  RightPortType=output  PseudoPeriodic=off  Frequencies=[]  NoiseDistribution=none  NoiseParameters=[]  Unit=1  AffineConversion=off  FilteringAndDerivatives=provide  SimscapeFilterOrder=1  InputFilterTimeConstant=0.001  UdotUserProvided=0
  P : PMIOPort  Side=Left
  N : PMIOPort  Port=2  Side=Right
  wires:
  g/1 -> Simulink-PS Converter/1
  connections:
  SPST Switch/LConn2 -- Capacitor/LConn1 -- P/RConn1
  Simulink-PS Converter/RConn1 -- SPST Switch/LConn1
  SPST Switch/RConn1 -- Resistor/RConn1 -- N/RConn1
  Capacitor/RConn1 -- Resistor/LConn1

== system simetran/MATE_SSE_3Level (3ph)/MATE_SSC_3Level2/Subsystem1 ==
  g : Inport
  Capacitor : fl_lib/Electrical/Electrical Elements/Capacitor  c=SnubberCapacitance F  r=0 Ohm  g=0 1/Ohm  i_specify=off  i_priority=None  i=0 A  i_nominal_specify=off  i_nominal_value=1  i_nominal_unit=A  v_specify=off  v_priority=None  v=0 V  v_nominal_specify=off  v_nominal_value=1  v_nominal_unit=V  vc_specify=off  vc_priority=High  vc=0 V  vc_nominal_specify=off  vc_nominal_value=1  vc_nominal_unit=V
  Resistor : fl_lib/Electrical/Electrical Elements/Resistor  R=SnubberResistance Ohm  i_specify=off  i_priority=None  i=0 A  i_nominal_specify=off  i_nominal_value=1  i_nominal_unit=A  v_specify=off  v_priority=None  v=0 V  v_nominal_specify=off  v_nominal_value=1  v_nominal_unit=V
  SPST Switch : ee_lib/Switches & Breakers/SPST Switch  R_closed=Ron*2 Ohm  G_open=1e-6 S  Threshold=0.5 V  Width=0 V  model_dynamics=0  t_on=1e-3 s  t_off=1e-3 s  initial_vT=0 V
      settings: InternalSimscapePortConfiguration="{\"Bottom\":[],\"Left\":[{\"id\":\"vT\",\"label\":\"vT\",\"type\":\"input\"},{\"id\":\"p\",\"label\":\"\",\"type\":\"foundation.electrical.electrical\"}],\"Right\":[{\"id\":\"n\",\"label\":\"\",\"type\":\"foundation.electrical.electrical\"}],\"Top\":[]}"
  Simulink-PS Converter : nesl_utility/Simulink-PS Converter  PhysicalDomain=network_engine_domain  SubClassName=ps_input  LeftPortType=input  RightPortType=output  PseudoPeriodic=off  Frequencies=[]  NoiseDistribution=none  NoiseParameters=[]  Unit=1  AffineConversion=off  FilteringAndDerivatives=provide  SimscapeFilterOrder=1  InputFilterTimeConstant=0.001  UdotUserProvided=0
  P : PMIOPort  Side=Left
  N : PMIOPort  Port=2  Side=Right
  wires:
  g/1 -> Simulink-PS Converter/1
  connections:
  SPST Switch/LConn2 -- Capacitor/LConn1 -- P/RConn1
  Simulink-PS Converter/RConn1 -- SPST Switch/LConn1
  SPST Switch/RConn1 -- Resistor/RConn1 -- N/RConn1
  Capacitor/RConn1 -- Resistor/LConn1

== system simetran/MATE_SSE_3Level (3ph)/MATE_SSC_3Level2/Subsystem2 ==
  g : Inport
  Capacitor : fl_lib/Electrical/Electrical Elements/Capacitor  c=SnubberCapacitance F  r=0 Ohm  g=0 1/Ohm  i_specify=off  i_priority=None  i=0 A  i_nominal_specify=off  i_nominal_value=1  i_nominal_unit=A  v_specify=off  v_priority=None  v=0 V  v_nominal_specify=off  v_nominal_value=1  v_nominal_unit=V  vc_specify=off  vc_priority=High  vc=0 V  vc_nominal_specify=off  vc_nominal_value=1  vc_nominal_unit=V
  Resistor : fl_lib/Electrical/Electrical Elements/Resistor  R=SnubberResistance Ohm  i_specify=off  i_priority=None  i=0 A  i_nominal_specify=off  i_nominal_value=1  i_nominal_unit=A  v_specify=off  v_priority=None  v=0 V  v_nominal_specify=off  v_nominal_value=1  v_nominal_unit=V
  SPST Switch : ee_lib/Switches & Breakers/SPST Switch  R_closed=Ron*2 Ohm  G_open=1e-6 S  Threshold=0.5 V  Width=0 V  model_dynamics=0  t_on=1e-3 s  t_off=1e-3 s  initial_vT=0 V
      settings: InternalSimscapePortConfiguration="{\"Bottom\":[],\"Left\":[{\"id\":\"vT\",\"label\":\"vT\",\"type\":\"input\"},{\"id\":\"p\",\"label\":\"\",\"type\":\"foundation.electrical.electrical\"}],\"Right\":[{\"id\":\"n\",\"label\":\"\",\"type\":\"foundation.electrical.electrical\"}],\"Top\":[]}"
  Simulink-PS Converter : nesl_utility/Simulink-PS Converter  PhysicalDomain=network_engine_domain  SubClassName=ps_input  LeftPortType=input  RightPortType=output  PseudoPeriodic=off  Frequencies=[]  NoiseDistribution=none  NoiseParameters=[]  Unit=1  AffineConversion=off  FilteringAndDerivatives=provide  SimscapeFilterOrder=1  InputFilterTimeConstant=0.001  UdotUserProvided=0
  P : PMIOPort  Side=Left
  N : PMIOPort  Port=2  Side=Right
  wires:
  g/1 -> Simulink-PS Converter/1
  connections:
  Capacitor/RConn1 -- Resistor/LConn1
  N/RConn1 -- Resistor/RConn1 -- SPST Switch/RConn1
  Simulink-PS Converter/RConn1 -- SPST Switch/LConn1
  P/RConn1 -- Capacitor/LConn1 -- SPST Switch/LConn2

== system simetran/MATE_SSE_3Level (3ph)/MATE_SSC_3Level3/Subsystem ==
  g : Inport
  Capacitor : fl_lib/Electrical/Electrical Elements/Capacitor  c=SnubberCapacitance F  r=0 Ohm  g=0 1/Ohm  i_specify=off  i_priority=None  i=0 A  i_nominal_specify=off  i_nominal_value=1  i_nominal_unit=A  v_specify=off  v_priority=None  v=0 V  v_nominal_specify=off  v_nominal_value=1  v_nominal_unit=V  vc_specify=off  vc_priority=High  vc=0 V  vc_nominal_specify=off  vc_nominal_value=1  vc_nominal_unit=V
  Resistor : fl_lib/Electrical/Electrical Elements/Resistor  R=SnubberResistance Ohm  i_specify=off  i_priority=None  i=0 A  i_nominal_specify=off  i_nominal_value=1  i_nominal_unit=A  v_specify=off  v_priority=None  v=0 V  v_nominal_specify=off  v_nominal_value=1  v_nominal_unit=V
  SPST Switch : ee_lib/Switches & Breakers/SPST Switch  R_closed=Ron*2 Ohm  G_open=1e-6 S  Threshold=0.5 V  Width=0 V  model_dynamics=0  t_on=1e-3 s  t_off=1e-3 s  initial_vT=0 V
      settings: InternalSimscapePortConfiguration="{\"Bottom\":[],\"Left\":[{\"id\":\"vT\",\"label\":\"vT\",\"type\":\"input\"},{\"id\":\"p\",\"label\":\"\",\"type\":\"foundation.electrical.electrical\"}],\"Right\":[{\"id\":\"n\",\"label\":\"\",\"type\":\"foundation.electrical.electrical\"}],\"Top\":[]}"
  Simulink-PS Converter : nesl_utility/Simulink-PS Converter  PhysicalDomain=network_engine_domain  SubClassName=ps_input  LeftPortType=input  RightPortType=output  PseudoPeriodic=off  Frequencies=[]  NoiseDistribution=none  NoiseParameters=[]  Unit=1  AffineConversion=off  FilteringAndDerivatives=provide  SimscapeFilterOrder=1  InputFilterTimeConstant=0.001  UdotUserProvided=0
  P : PMIOPort  Side=Left
  N : PMIOPort  Port=2  Side=Right
  wires:
  g/1 -> Simulink-PS Converter/1
  connections:
  SPST Switch/LConn2 -- Capacitor/LConn1 -- P/RConn1
  Simulink-PS Converter/RConn1 -- SPST Switch/LConn1
  SPST Switch/RConn1 -- Resistor/RConn1 -- N/RConn1
  Capacitor/RConn1 -- Resistor/LConn1

== system simetran/MATE_SSE_3Level (3ph)/MATE_SSC_3Level3/Subsystem1 ==
  g : Inport
  Capacitor : fl_lib/Electrical/Electrical Elements/Capacitor  c=SnubberCapacitance F  r=0 Ohm  g=0 1/Ohm  i_specify=off  i_priority=None  i=0 A  i_nominal_specify=off  i_nominal_value=1  i_nominal_unit=A  v_specify=off  v_priority=None  v=0 V  v_nominal_specify=off  v_nominal_value=1  v_nominal_unit=V  vc_specify=off  vc_priority=High  vc=0 V  vc_nominal_specify=off  vc_nominal_value=1  vc_nominal_unit=V
  Resistor : fl_lib/Electrical/Electrical Elements/Resistor  R=SnubberResistance Ohm  i_specify=off  i_priority=None  i=0 A  i_nominal_specify=off  i_nominal_value=1  i_nominal_unit=A  v_specify=off  v_priority=None  v=0 V  v_nominal_specify=off  v_nominal_value=1  v_nominal_unit=V
  SPST Switch : ee_lib/Switches & Breakers/SPST Switch  R_closed=Ron*2 Ohm  G_open=1e-6 S  Threshold=0.5 V  Width=0 V  model_dynamics=0  t_on=1e-3 s  t_off=1e-3 s  initial_vT=0 V
      settings: InternalSimscapePortConfiguration="{\"Bottom\":[],\"Left\":[{\"id\":\"vT\",\"label\":\"vT\",\"type\":\"input\"},{\"id\":\"p\",\"label\":\"\",\"type\":\"foundation.electrical.electrical\"}],\"Right\":[{\"id\":\"n\",\"label\":\"\",\"type\":\"foundation.electrical.electrical\"}],\"Top\":[]}"
  Simulink-PS Converter : nesl_utility/Simulink-PS Converter  PhysicalDomain=network_engine_domain  SubClassName=ps_input  LeftPortType=input  RightPortType=output  PseudoPeriodic=off  Frequencies=[]  NoiseDistribution=none  NoiseParameters=[]  Unit=1  AffineConversion=off  FilteringAndDerivatives=provide  SimscapeFilterOrder=1  InputFilterTimeConstant=0.001  UdotUserProvided=0
  P : PMIOPort  Side=Left
  N : PMIOPort  Port=2  Side=Right
  wires:
  g/1 -> Simulink-PS Converter/1
  connections:
  SPST Switch/LConn2 -- Capacitor/LConn1 -- P/RConn1
  Simulink-PS Converter/RConn1 -- SPST Switch/LConn1
  SPST Switch/RConn1 -- Resistor/RConn1 -- N/RConn1
  Capacitor/RConn1 -- Resistor/LConn1

== system simetran/MATE_SSE_3Level (3ph)/MATE_SSC_3Level3/Subsystem2 ==
  g : Inport
  Capacitor : fl_lib/Electrical/Electrical Elements/Capacitor  c=SnubberCapacitance F  r=0 Ohm  g=0 1/Ohm  i_specify=off  i_priority=None  i=0 A  i_nominal_specify=off  i_nominal_value=1  i_nominal_unit=A  v_specify=off  v_priority=None  v=0 V  v_nominal_specify=off  v_nominal_value=1  v_nominal_unit=V  vc_specify=off  vc_priority=High  vc=0 V  vc_nominal_specify=off  vc_nominal_value=1  vc_nominal_unit=V
  Resistor : fl_lib/Electrical/Electrical Elements/Resistor  R=SnubberResistance Ohm  i_specify=off  i_priority=None  i=0 A  i_nominal_specify=off  i_nominal_value=1  i_nominal_unit=A  v_specify=off  v_priority=None  v=0 V  v_nominal_specify=off  v_nominal_value=1  v_nominal_unit=V
  SPST Switch : ee_lib/Switches & Breakers/SPST Switch  R_closed=Ron*2 Ohm  G_open=1e-6 S  Threshold=0.5 V  Width=0 V  model_dynamics=0  t_on=1e-3 s  t_off=1e-3 s  initial_vT=0 V
      settings: InternalSimscapePortConfiguration="{\"Bottom\":[],\"Left\":[{\"id\":\"vT\",\"label\":\"vT\",\"type\":\"input\"},{\"id\":\"p\",\"label\":\"\",\"type\":\"foundation.electrical.electrical\"}],\"Right\":[{\"id\":\"n\",\"label\":\"\",\"type\":\"foundation.electrical.electrical\"}],\"Top\":[]}"
  Simulink-PS Converter : nesl_utility/Simulink-PS Converter  PhysicalDomain=network_engine_domain  SubClassName=ps_input  LeftPortType=input  RightPortType=output  PseudoPeriodic=off  Frequencies=[]  NoiseDistribution=none  NoiseParameters=[]  Unit=1  AffineConversion=off  FilteringAndDerivatives=provide  SimscapeFilterOrder=1  InputFilterTimeConstant=0.001  UdotUserProvided=0
  P : PMIOPort  Side=Left
  N : PMIOPort  Port=2  Side=Right
  wires:
  g/1 -> Simulink-PS Converter/1
  connections:
  Capacitor/RConn1 -- Resistor/LConn1
  N/RConn1 -- Resistor/RConn1 -- SPST Switch/RConn1
  Simulink-PS Converter/RConn1 -- SPST Switch/LConn1
  P/RConn1 -- Capacitor/LConn1 -- SPST Switch/LConn2

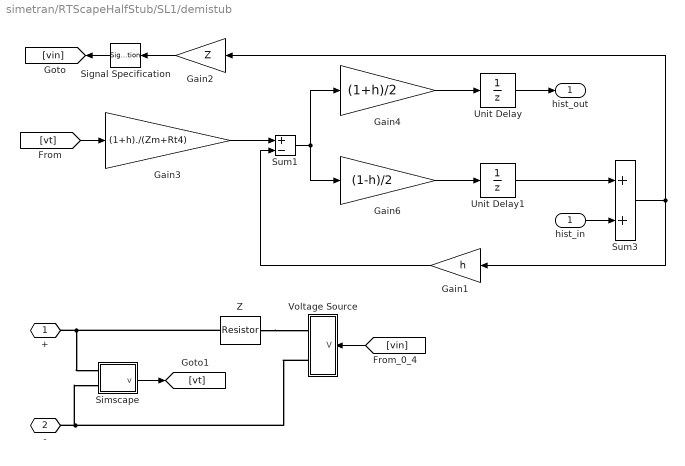
== system simetran/RTScapeHalfStub/SL1/demistub ==
  hist_in : Inport
  Gain1 : Gain  Gain=h  SaturateOnIntegerOverflow=on  OutDataTypeStr=Inherit: Same as input  ParamDataTypeStr=Inherit: Same as input
  Gain2 : Gain  Gain=Z  SaturateOnIntegerOverflow=on  OutDataTypeStr=Inherit: Same as input  ParamDataTypeStr=Inherit: Same as input
  Gain3 : Gain  Gain=(1+h)./(Zm+Rt4)  SaturateOnIntegerOverflow=on  OutDataTypeStr=Inherit: Same as input  ParamDataTypeStr=Inherit: Same as input
  Gain4 : Gain  Gain=(1+h)/2  SaturateOnIntegerOverflow=on  OutDataTypeStr=Inherit: Same as input  ParamDataTypeStr=Inherit: Same as input
  Gain6 : Gain  Gain=(1-h)/2  SaturateOnIntegerOverflow=on  OutDataTypeStr=Inherit: Same as input  ParamDataTypeStr=Inherit: Same as input
  Signal Specification : SignalSpecification  Dimensions=1
  Simscape : Subsystem
      mask Display: disp('V')
  Sum1 : Sum  Inputs=+-  InputSameDT=on  SaturateOnIntegerOverflow=on  OutDataTypeStr=Inherit: Same as first input
  Sum3 : Sum  InputSameDT=on  SaturateOnIntegerOverflow=on  OutDataTypeStr=Inherit: Same as first input
  Unit Delay : UnitDelay  SampleTime=Ts  HasFrameUpgradeWarning=on
  Unit Delay1 : UnitDelay  SampleTime=Ts  HasFrameUpgradeWarning=on
  Voltage Source : Subsystem
  Z : ee_lib/Passive/Resistor  R=Z Ohm  enable_R_tol=ee.enum.toleranceApplication.none  R_tol=5  tol_distribution=ee.enum.toleranceDistribution.uniform  nSigma=4  enable_operating_limits=ee.enum.enable.no  operating_limit_action=ee.enum.passive.reportOpLim.warn  power_rating=1 W  max_working_voltage=100 V  noise_mode=ee.enum.sources.noise.Disabled  Tdevice=25 degC  sample_time=1e-3 s  repeatability=ee.enum.ic.repeatability.notRepeatable  user_seed=0  auto_seed=153380492  fault_action=simscape.enum.assert.action.none  t_fault=1 s  power_derating_T1=70 degC  power_derating_T2=155 degC  operating_temperature_range_vec=[-50, 150] degC  alpha=3.93e-3 1/K  Tmeas=25 degC  thermal_mass=100 J/K  temperature_specify=off  temperature_priority=High  temperature=298.15 K  temperature_nominal_specify=off  temperature_nominal_value=1  temperature_nominal_unit=K
  + : PMIOPort  Side=Left
  - : PMIOPort  Port=2  Side=Left
  hist_out : Outport  VectorParamsAs1DForOutWhenUnconnected=off
  wires:
  Unit Delay1/1 -> Sum3/1
  Unit Delay/1 -> hist_out/1
  hist_in/1 -> Sum3/2
  Gain2/1 -> Signal Specification/1
  Sum3/1 -> Gain2/1, Gain1/1
  Gain4/1 -> Unit Delay/1
  Gain6/1 -> Unit Delay1/1
  Sum1/1 -> Gain6/1, Gain4/1
  [vin] -> Voltage Source/1(V)
  Signal Specification/1 -> [vin]
  Simscape/1(v) -> [vt]
  [vt] -> Gain3/1
  Gain3/1 -> Sum1/1
  Gain1/1 -> Sum1/2
  connections:
  Voltage Source/RConn2 -- Simscape/LConn2 -- -/RConn1
  Z/LConn1 -- Voltage Source/RConn1
  Z/RConn1 -- Simscape/LConn1 -- +/RConn1

== system simetran/RTScapeHalfStub/SL1/demistub/Simscape ==
  PS-S : nesl_utility/PS-Simulink Converter  PhysicalDomain=network_engine_domain  SubClassName=ps_output  LeftPortType=input  RightPortType=output  PseudoPeriodic=off  Frequencies=[]  VectorFormat=1-D array  Unit=V  AffineConversion=off
  Voltage Sensor : fl_lib/Electrical/Electrical Sensors/Voltage Sensor
  V+ : PMIOPort  Side=Left
  V- : PMIOPort  Port=2  Side=Left
  v : Outport  VectorParamsAs1DForOutWhenUnconnected=off
  wires:
  PS-S/1 -> v/1  "voltage"
  connections:
  V-/RConn1 -- Voltage Sensor/RConn2
  V+/RConn1 -- Voltage Sensor/LConn1
  PS-S/LConn1 -- Voltage Sensor/RConn1
